simulink model "xiti4_8_10"  (Simulink 8.3)
settings: Solver=ode45  StartTime=0.0  StopTime=200  FixedStep=0.01  RelTol=1e-3
libraries: simulink_need_slupdate x6
CloseFcn:
  | rtwprivate ssgensfun ModelCloseRequest PID_PI
settings Model: Creator=sony  LastModifiedBy=sony
settings DataIOCC: SignalLoggingName=sigsOut
settings DebuggingCC: SaveWithParameterizedLinksMsg=none  SignalResolutionControl=TryResolveAllWithWarning  SolverPrmCheckMsg=none  MultiTaskDSMMsg=warning  MultiTaskCondExecSysMsg=none  StateNameClashWarn=none
settings HardwareCC: TargetUnknown=on
settings RTWCC: IncludeERTFirstTime=on

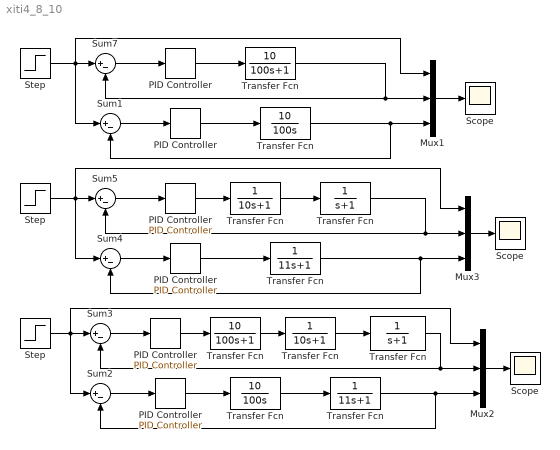
== system xiti4_8_10 ==
  "  PID Controller " : simulink_need_slupdate/PID Controller  P=3  I=0  D=0
  "  Transfer Fcn" : TransferFcn  Denominator=[1 1]
  "  Transfer Fcn " : TransferFcn  Denominator=[1 1]
  "  Transfer Fcn  " : TransferFcn  Numerator=[10]  Denominator=[100 1]
  "  Transfer Fcn   " : TransferFcn  Denominator=[11 1]
  " PID Controller" : simulink_need_slupdate/PID Controller  P=1  I=0  D=0
  " PID Controller " : simulink_need_slupdate/PID Controller  P=1  I=0  D=0
  " PID Controller   " : simulink_need_slupdate/PID Controller  P=3  I=0  D=0
  " Scope " : Scope
      settings: TimeRange=300  YMin=0  YMax=1.4  SaveName=xiti4_83  MaxDataPoints=500000
  " Transfer Fcn  " : TransferFcn  Denominator=[11 1]
  " Transfer Fcn   " : TransferFcn  Denominator=[10 1]
  Mux1 : Mux  Inputs=3
  Mux2 : Mux  Inputs=3
  Mux3 : Mux  Inputs=3
  PID Controller : simulink_need_slupdate/PID Controller  P=10  I=0  D=0
  "PID Controller " : simulink_need_slupdate/PID Controller  P=10  I=0  D=0
  Scope : Scope
      settings: TimeRange=20.2729044834308  YMin=0.36128  YMax=0.809451  SaveName=xiti4_82  MaxDataPoints=500000
  "Scope " : Scope
      settings: YMin=0  YMax=1.5  SaveName=xiti4_81  MaxDataPoints=500000
  Step : Step  Time=0  SampleTime=0
  "Step " : Step  Time=0  SampleTime=0
  "Step  " : Step  Time=0  SampleTime=0
  Sum{1..5,7} (6 alike) : Sum  Inputs=|+-  SaturateOnIntegerOverflow=on
  Transfer Fcn : TransferFcn  Numerator=[10]  Denominator=[100 1]
  "Transfer Fcn " : TransferFcn  Numerator=[10]  Denominator=[100 0]
  "Transfer Fcn  " : TransferFcn  Denominator=[10 1]
  "Transfer Fcn   " : TransferFcn  Numerator=[10]  Denominator=[100 0]
  wires:
  Step/1 -> Sum7/1, Sum1/1, Mux1/1
  Sum7/1 -> "PID Controller "/1
  "PID Controller "/1 -> Transfer Fcn/1
  Transfer Fcn/1 -> Sum7/2, Mux1/2
  Sum1/1 -> PID Controller/1
  PID Controller/1 -> "Transfer Fcn "/1
  "Transfer Fcn "/1 -> Sum1/2, Mux1/3
  Mux1/1 -> "Scope "/1
  "Step  "/1 -> Sum3/1, Mux2/1, Sum2/1
  Sum3/1 -> "  PID Controller "/1
  "  PID Controller "/1 -> "  Transfer Fcn  "/1
  " Transfer Fcn   "/1 -> "  Transfer Fcn"/1
  Sum2/1 -> " PID Controller   "/1
  " PID Controller   "/1 -> "Transfer Fcn   "/1
  Mux2/1 -> " Scope "/1
  "  Transfer Fcn"/1 -> Sum3/2, Mux2/2
  "  Transfer Fcn  "/1 -> " Transfer Fcn   "/1
  "  Transfer Fcn   "/1 -> Sum2/2, Mux2/3
  "Transfer Fcn   "/1 -> "  Transfer Fcn   "/1
  "Step "/1 -> Sum5/1, Sum4/1, Mux3/1
  Sum5/1 -> " PID Controller "/1
  " PID Controller "/1 -> "Transfer Fcn  "/1
  "Transfer Fcn  "/1 -> "  Transfer Fcn "/1
  Sum4/1 -> " PID Controller"/1
  " PID Controller"/1 -> " Transfer Fcn  "/1
  Mux3/1 -> Scope/1
  "  Transfer Fcn "/1 -> Sum5/2, Mux3/2
  " Transfer Fcn  "/1 -> Sum4/2, Mux3/3
